simulink subsystem "Baseline"  (R2025b)
settings: Solver=VariableStepAuto  StartTime=0.0  StopTime=10.0  RelTol=1e-3
undefined symbols (not defined in the file): As_lat, As_lon, L1_LPF_bw, SimIn, SimPar, useL1
libraries: simulink_extras x23, ComponentsLib x11, matrix_library x2, AdaptiveLib x1, libAxisTransformations x1
settings Model: Creator=tbritton  LastModifiedBy=bullo
settings SolverCC: AlgebraicLoopSolver=TrustRegion
settings OptimizationCC: ReuseModelBlockBuffer=off
settings DebuggingCC: UnconnectedInputMsg=warning  UnconnectedOutputMsg=warning  UnconnectedLineMsg=warning
settings ModelReferenceCC: EnableRefExpFcnMdlSchedulingChecks=on
settings RTWCC: GPUComputeCapability=3.5  DLArmComputeVersion=19.05

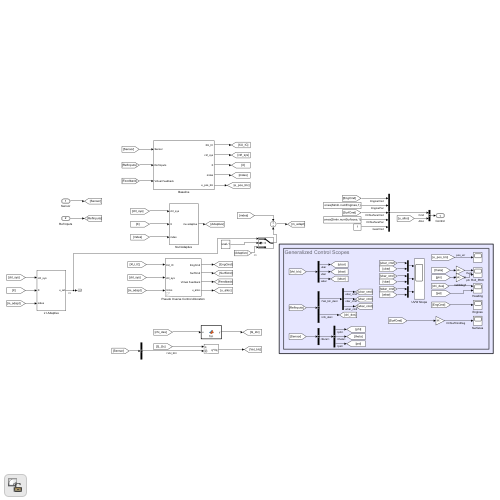
[thumbnail: Simulink's stored preview of the top-level diagram]
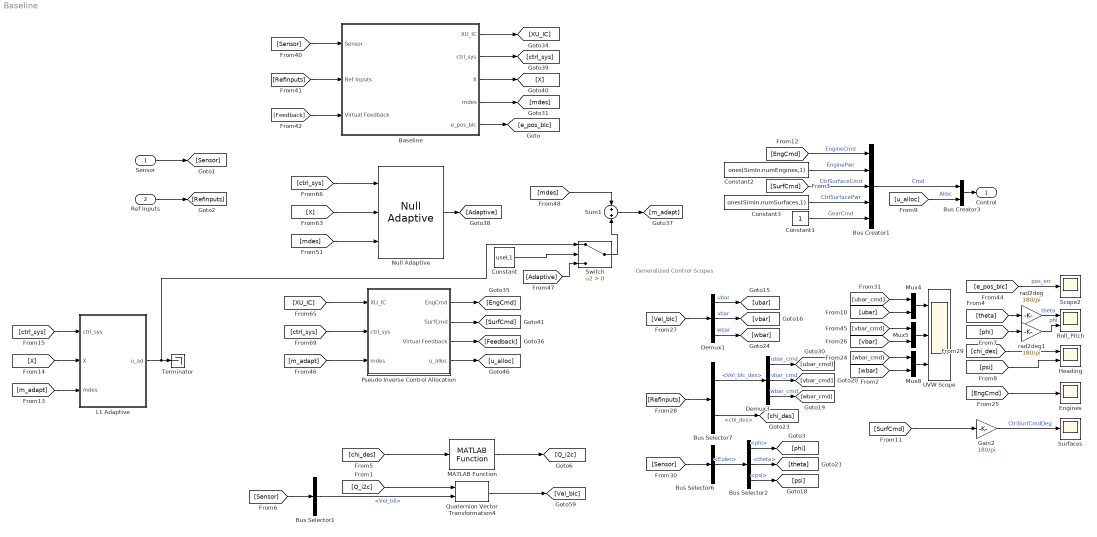
== system Baseline ==
  note: Generalized Control Scopes
  Sensor : Inport  OutDataTypeStr=Bus: SensorBus
  Ref Inputs : Inport  Port=2  OutDataTypeStr=Bus: BUS_REF_INPUT
  Baseline : Subsystem
      settings: LibrarySourceBlock=ControllersLib/Baseline
  Bus Creator1 : BusCreator  Inputs=5  OutDataTypeStr=Bus: BUS_CMD
  Bus Creator3 : BusCreator  Inputs=2
  Bus Selector1 : BusSelector  OutputSignals=Vel_bIi
  Bus Selector2 : BusSelector  OutputSignals=phi,theta,psi
  Bus Selector6 : BusSelector  OutputSignals=Euler
  Bus Selector7 : BusSelector  OutputSignals=Vel_bIc_des,chi_des
  Constant : Constant  Value=useL1
  Constant1 : Constant
  Constant2 : Constant  Value=ones(SimIn.numEngines,1)
  Constant3 : Constant  Value=ones(SimIn.numSurfaces,1)
  Demux1 : Demux  Outputs=3
  Demux3 : Demux  Outputs=3
  Engines : Scope
      settings: ActiveDisplayYMinimum=-12.285  ActiveDisplayYMaximum=110.56496
  Gain2 : Gain  Gain=180/pi
  Heading : Scope  NumInputPorts=2
      settings: ActiveDisplayYMinimum=-1.5E-19  ActiveDisplayYMaximum=1.3E-19  DataLoggingVariableName=ScopeData2
  L1 Adaptive : Subsystem
  MATLAB Function : ComponentsLib/ConvertToControlFrame/MATLAB Function  SystemSampleTime=-1  VariantActivationTime=update diagram  EmptyChoice=off  PassThrough=off  PassThroughVariantControl=(default)  EmptyChoiceVariantControl=(default)  AllowFlexibleInterface=on  Latency=0  AutoFrameSizeCalculation=off
      settings: SourceProductName=Components
  Mux4 : Mux  Inputs=2
  Mux5 : Mux  Inputs=2
  Mux8 : Mux  Inputs=2
  Null Adaptive : AdaptiveLib/Null Adaptive  SystemSampleTime=-1  VariantActivationTime=update diagram  EmptyChoice=off  PassThrough=off  PassThroughVariantControl=(default)  EmptyChoiceVariantControl=(default)  AllowFlexibleInterface=on  Latency=0  AutoFrameSizeCalculation=off
      settings: SourceProductName=Adaptive Augmentation
  Pseudo Inverse Control Allocation : Subsystem  AncestorBlock=AllocatorsLib/Pseudo Inverse Control Allocation
      settings: LibrarySourceBlock=AllocatorsLib/Pseudo Inverse Control Allocation
  Quaternion Vector Transformation4 : libAxisTransformations/Quaternion Vector Transformation  n=0
  Roll_Pitch : Scope  NumInputPorts=2
      settings: ActiveDisplayYMinimum=-0.0002  ActiveDisplayYMaximum=0.00013  DataLoggingVariableName=ScopeData3
  Scope2 : Scope
      settings: ActiveDisplayYMinimum=-0.07649  ActiveDisplayYMaximum=0.00878  DataLoggingVariableName=ScopeData4
  Sum1 : Sum
  Surfaces : Scope
      settings: ActiveDisplayYMinimum=-0.05034  ActiveDisplayYMaximum=0.00559  DataLoggingVariableName=ScopeData5
  Switch : Switch  Criteria=u2 > Threshold  SaturateOnIntegerOverflow=off  InputSameDT=off
  Terminator : Terminator
  UVW Scope : Scope  NumInputPorts=3
      settings: Title=UVW Commands vs Actual  ActiveDisplayYMinimum=-0.00149  ActiveDisplayYMaximum=0.01337  DataLoggingVariableName=ScopeData6
  rad2deg : Gain  Gain=180/pi
  rad2deg1 : Gain  Gain=180/pi
  Control : Outport  OutDataTypeStr=Bus: BUS_CONTROL  VectorParamsAs1DForOutWhenUnconnected=off
  wires:
  rad2deg1/1 -> Roll_Pitch/2  "phi"
  rad2deg/1 -> Roll_Pitch/1  "theta"
  Ref Inputs/1 -> [RefInputs]
  [u_alloc] -> Bus Creator3/2  "Alloc"
  Bus Creator3/1 -> Control/1
  Constant1/1 -> Bus Creator1/5  "GearCmd"
  [SurfCmd] -> Bus Creator1/3  "CtrlSurfaceCmd"
  Bus Creator1/1 -> Bus Creator3/1  "Cmd"
  Sensor/1 -> [Sensor]
  [EngCmd] -> Bus Creator1/1  "EngineCmd"
  Constant2/1 -> Bus Creator1/2  "EnginePwr"
  Constant3/1 -> Bus Creator1/4  "CtrlSurfacePwr"
  [Sensor] -> Baseline/1(Sensor)
  [RefInputs] -> Baseline/2(Ref Inputs)
  [Feedback] -> Baseline/3(Virtual Feedback)
  Baseline/4(mdes) -> [mdes]
  [m_adapt] -> Pseudo Inverse Control Allocation/3(mdes)
  Pseudo Inverse Control Allocation/3(Virtual Feedback) -> [Feedback]
  Baseline/1(XU_IC) -> [XU_IC]
  Pseudo Inverse Control Allocation/1(EngCmd) -> [EngCmd]
  [ctrl_sys] -> Null Adaptive/1
  [mdes] -> Null Adaptive/3
  [X] -> Null Adaptive/2
  Null Adaptive/1 -> [Adaptive]
  Baseline/2(ctrl_sys) -> [ctrl_sys]
  Baseline/3(X) -> [X]
  Sum1/1 -> [m_adapt]
  [mdes] -> Sum1/1
  Pseudo Inverse Control Allocation/2(SurfCmd) -> [SurfCmd]
  Pseudo Inverse Control Allocation/4(u_alloc) -> [u_alloc]
  [XU_IC] -> Pseudo Inverse Control Allocation/1(XU_IC)
  [ctrl_sys] -> Pseudo Inverse Control Allocation/2(ctrl_sys)
  Bus Selector1/1 -> Quaternion Vector Transformation4/2  "<Vel_bIi>"
  [Q_i2c] -> Quaternion Vector Transformation4/1
  [chi_des] -> MATLAB Function/1
  Quaternion Vector Transformation4/1 -> [Vel_bIc]
  MATLAB Function/1 -> [Q_i2c]
  [Sensor] -> Bus Selector1/1
  Demux1/3 -> [wbar]  "wbar"
  [wbar_cmd] -> Mux8/1
  Bus Selector7/2 -> [chi_des]  "<chi_des>"
  [Vel_bIc] -> Demux1/1
  Demux3/1 -> [ubar_cmd]  "ubar_cmd"
  Bus Selector7/1 -> Demux3/1  "<Vel_bIc_des>"
  [EngCmd] -> Engines/1
  Demux1/2 -> [vbar]  "vbar"
  [psi] -> Heading/2
  Bus Selector2/2 -> [theta]  "<theta>"
  [theta] -> rad2deg/1
  Gain2/1 -> Surfaces/1  "CtrlSurfCmdDeg"
  Bus Selector2/3 -> [psi]  "<psi>"
  Mux8/1 -> UVW Scope/3
  Bus Selector2/1 -> [phi]  "<phi>"
  Bus Selector6/1 -> Bus Selector2/1  "<Euler>"
  [e_pos_bIc] -> Scope2/1  "pos_err"
  Demux3/2 -> [vbar_cmd]  "vbar_cmd"
  [phi] -> rad2deg1/1
  [wbar] -> Mux8/2
  [RefInputs] -> Bus Selector7/1
  [Sensor] -> Bus Selector6/1
  [ubar] -> Mux4/2
  [chi_des] -> Heading/1
  [SurfCmd] -> Gain2/1
  [vbar] -> Mux5/2
  [ubar_cmd] -> Mux4/1
  [vbar_cmd] -> Mux5/1
  Mux5/1 -> UVW Scope/2
  Demux3/3 -> [wbar_cmd]  "wbar_cmd"
  Mux4/1 -> UVW Scope/1
  Demux1/1 -> [ubar]  "ubar"
  Baseline/5(e_pos_blc) -> [e_pos_bIc]
  [ctrl_sys] -> L1 Adaptive/1(ctrl_sys)
  [X] -> L1 Adaptive/2(X)
  [m_adapt] -> L1 Adaptive/3(mdes)
  Switch/1 -> Sum1/2
  L1 Adaptive/1(u_ad) -> Terminator/1, Switch/1
  [Adaptive] -> Switch/3
  Constant/1 -> Switch/2

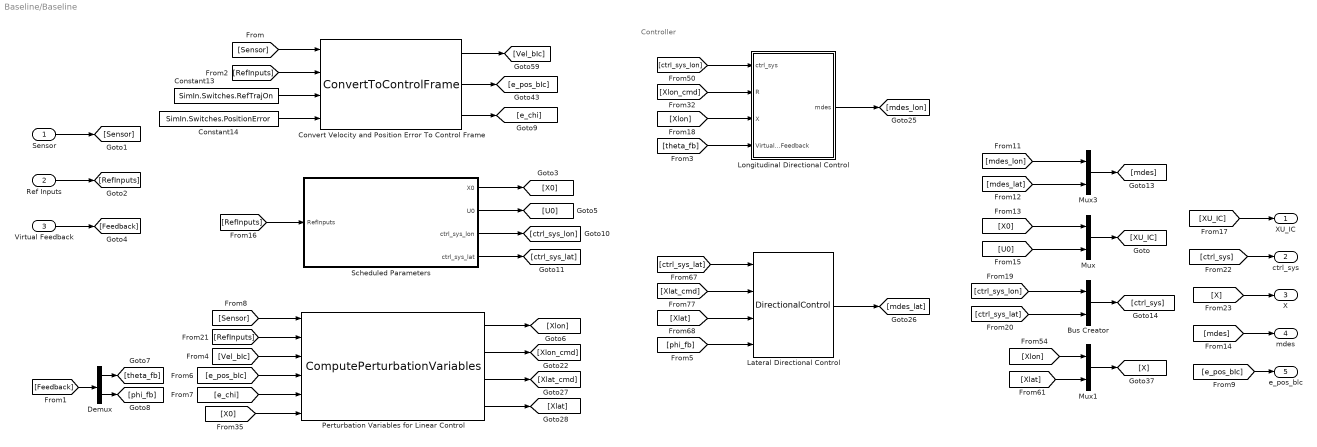
== system Baseline/Baseline ==
  note: Controller
  Sensor : Inport  OutDataTypeStr=Bus: SensorBus
  Ref Inputs : Inport  Port=2  OutDataTypeStr=Bus: BUS_REF_INPUT
  Virtual Feedback : Inport  Port=3
  Bus Creator : BusCreator  Inputs=2
  Constant13 : Constant  Value=SimIn.Switches.RefTrajOn
  Constant14 : Constant  Value=SimIn.Switches.PositionError
  Convert Velocity and Position Error To Control Frame : ComponentsLib/ConvertToControlFrame  SystemSampleTime=-1  VariantActivationTime=update diagram  EmptyChoice=off  PassThrough=off  PassThroughVariantControl=(default)  EmptyChoiceVariantControl=(default)  AllowFlexibleInterface=on  Latency=0  AutoFrameSizeCalculation=off
      link override delta_cos: Inputs=|++
      settings: SourceProductName=Components
  Demux : Demux  Outputs=2
  Lateral Directional Control : ComponentsLib/DirectionalControl  SystemSampleTime=-1  VariantActivationTime=update diagram  EmptyChoice=off  PassThrough=off  PassThroughVariantControl=(default)  EmptyChoiceVariantControl=(default)  AllowFlexibleInterface=on  Latency=0  AutoFrameSizeCalculation=off
      settings: SourceProductName=Components
  Longitudinal Directional Control : Subsystem  AncestorBlock=ComponentsLib/DirectionalControl
      settings: LibrarySourceBlock=ComponentsLib/DirectionalControl
  Mux : Mux  Inputs=2
  Mux1 : Mux  Inputs=2
  Mux3 : Mux  Inputs=2
  Perturbation Variables for Linear Control : ComponentsLib/ComputePerturbationVariables  SystemSampleTime=-1  VariantActivationTime=update diagram  EmptyChoice=off  PassThrough=off  PassThroughVariantControl=(default)  EmptyChoiceVariantControl=(default)  AllowFlexibleInterface=on  Latency=0  AutoFrameSizeCalculation=off
      settings: SourceProductName=Components
  Scheduled Parameters : Subsystem  AncestorBlock=ComponentsLib/FeedbackScheduling
      settings: LibrarySourceBlock=ComponentsLib/FeedbackScheduling
  XU_IC : Outport
  ctrl_sys : Outport  Port=2
  X : Outport  Port=3
  mdes : Outport  Port=4
  e_pos_blc : Outport  Port=5
  wires:
  [mdes_lat] -> Mux3/2
  [e_pos_bIc] -> e_pos_blc/1
  [X0] -> Perturbation Variables for Linear Control/6
  Perturbation Variables for Linear Control/1 -> [Xlon]
  [Sensor] -> Perturbation Variables for Linear Control/1
  Perturbation Variables for Linear Control/3 -> [Xlat_cmd]
  Sensor/1 -> [Sensor]
  Scheduled Parameters/1(X0) -> [X0]
  Ref Inputs/1 -> [RefInputs]
  [RefInputs] -> Convert Velocity and Position Error To Control Frame/2
  Convert Velocity and Position Error To Control Frame/1 -> [Vel_bIc]
  Convert Velocity and Position Error To Control Frame/2 -> [e_pos_bIc]
  Scheduled Parameters/3(ctrl_sys_lon) -> [ctrl_sys_lon]
  [e_pos_bIc] -> Perturbation Variables for Linear Control/4
  Perturbation Variables for Linear Control/4 -> [Xlat]
  [RefInputs] -> Scheduled Parameters/1(RefInputs)
  Perturbation Variables for Linear Control/2 -> [Xlon_cmd]
  Convert Velocity and Position Error To Control Frame/3 -> [e_chi]
  [Sensor] -> Convert Velocity and Position Error To Control Frame/1
  [Vel_bIc] -> Perturbation Variables for Linear Control/3
  Constant13/1 -> Convert Velocity and Position Error To Control Frame/3
  [RefInputs] -> Perturbation Variables for Linear Control/2
  Constant14/1 -> Convert Velocity and Position Error To Control Frame/4
  [e_chi] -> Perturbation Variables for Linear Control/5
  Scheduled Parameters/2(U0) -> [U0]
  Scheduled Parameters/4(ctrl_sys_lat) -> [ctrl_sys_lat]
  [Xlon_cmd] -> Longitudinal Directional Control/2(R)
  Lateral Directional Control/1 -> [mdes_lat]
  [ctrl_sys_lat] -> Lateral Directional Control/1
  [ctrl_sys_lon] -> Longitudinal Directional Control/1(ctrl_sys)
  Longitudinal Directional Control/1(mdes) -> [mdes_lon]
  [Xlat] -> Lateral Directional Control/3
  [Xlon] -> Longitudinal Directional Control/3(X)
  [Xlat_cmd] -> Lateral Directional Control/2
  Virtual Feedback/1 -> [Feedback]
  [Feedback] -> Demux/1
  Demux/2 -> [phi_fb]
  Demux/1 -> [theta_fb]
  [theta_fb] -> Longitudinal Directional Control/4(Virtual Feedback)
  [phi_fb] -> Lateral Directional Control/4
  [mdes_lon] -> Mux3/1
  Mux3/1 -> [mdes]
  [mdes] -> mdes/1
  [X0] -> Mux/1
  [U0] -> Mux/2
  Mux/1 -> [XU_IC]
  [XU_IC] -> XU_IC/1
  [ctrl_sys_lon] -> Bus Creator/1
  [ctrl_sys_lat] -> Bus Creator/2
  Bus Creator/1 -> [ctrl_sys]
  [ctrl_sys] -> ctrl_sys/1
  Mux1/1 -> [X]
  [Xlon] -> Mux1/1
  [Xlat] -> Mux1/2
  [X] -> X/1

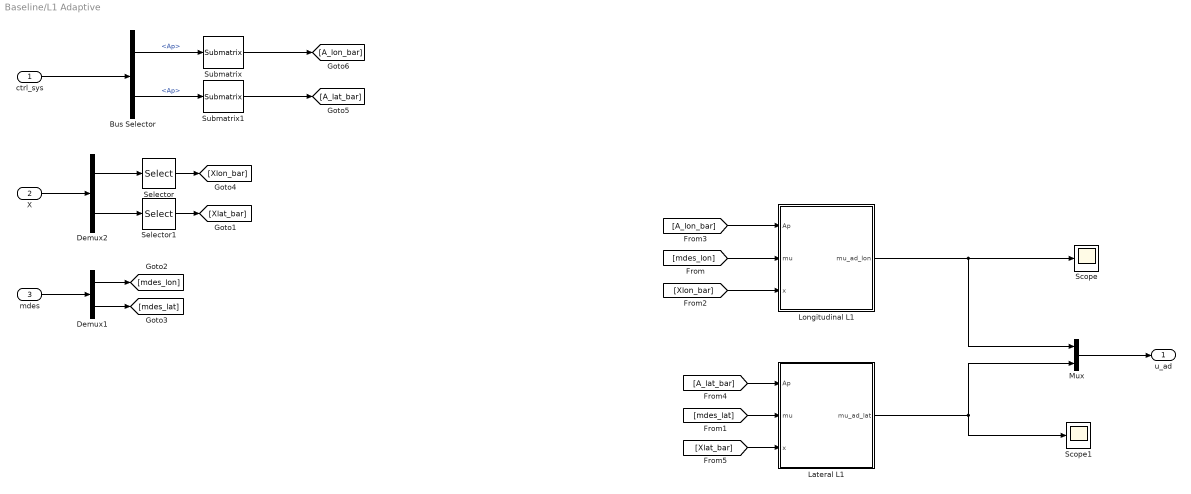
== system Baseline/L1 Adaptive ==
  ctrl_sys : Inport
  X : Inport  Port=2
  mdes : Inport  Port=3
  Bus Selector : BusSelector  OutputSignals=ctrl_sys_lon.Ap,ctrl_sys_lat.Ap
  Demux1 : Demux  Outputs=2
  Demux2 : Demux  Outputs=2
  Lateral L1 : Subsystem
  Longitudinal L1 : Subsystem
  Mux : Mux  Inputs=2
  Scope : Scope
      settings: ActiveDisplayYMinimum=-28.653376780680318  ActiveDisplayYMaximum=12.641940394712167  DataLoggingVariableName=ScopeData11
  Scope1 : Scope
      settings: ActiveDisplayYMinimum=-8.3781527224197525  ActiveDisplayYMaximum=15.883080645115539  DataLoggingVariableName=ScopeData12
  Selector : Selector  InputPortWidth=4  IndexOptions=Index vector (dialog)  Indices=[1:3]  OutputSizes=1
  Selector1 : Selector  InputPortWidth=4  IndexOptions=Index vector (dialog)  Indices=[1:3]  OutputSizes=1
  Submatrix : matrix_library/Submatrix  RowSpan=Range of rows  RowStartMode=First  RowStartIndex=1  RowEndMode=Index  RowEndIndex=3  ColSpan=Range of columns  ColStartMode=First  ColStartIndex=1  ColEndMode=Index  ColEndIndex=3
  Submatrix1 : matrix_library/Submatrix  RowSpan=Range of rows  RowStartMode=First  RowStartIndex=1  RowEndMode=Index  RowEndIndex=3  ColSpan=Range of columns  ColStartMode=First  ColStartIndex=1  ColEndMode=Index  ColEndIndex=3
  u_ad : Outport
  wires:
  [A_lat_bar] -> Lateral L1/1(Ap)
  [mdes_lat] -> Lateral L1/2(mu)
  Lateral L1/1(mu_ad_lat) -> Mux/2, Scope1/1
  [Xlat_bar] -> Lateral L1/3(x)
  [A_lon_bar] -> Longitudinal L1/1(Ap)
  Submatrix/1 -> [A_lon_bar]
  Submatrix1/1 -> [A_lat_bar]
  Bus Selector/2 -> Submatrix1/1  "<Ap>"
  Selector1/1 -> [Xlat_bar]
  [Xlon_bar] -> Longitudinal L1/3(x)
  Selector/1 -> [Xlon_bar]
  Mux/1 -> u_ad/1
  [mdes_lon] -> Longitudinal L1/2(mu)
  Longitudinal L1/1(mu_ad_lon) -> Scope/1, Mux/1
  Demux2/2 -> Selector1/1
  Demux2/1 -> Selector/1
  Bus Selector/1 -> Submatrix/1  "<Ap>"
  Demux1/1 -> [mdes_lon]
  Demux1/2 -> [mdes_lat]
  mdes/1 -> Demux1/1
  X/1 -> Demux2/1
  ctrl_sys/1 -> Bus Selector/1

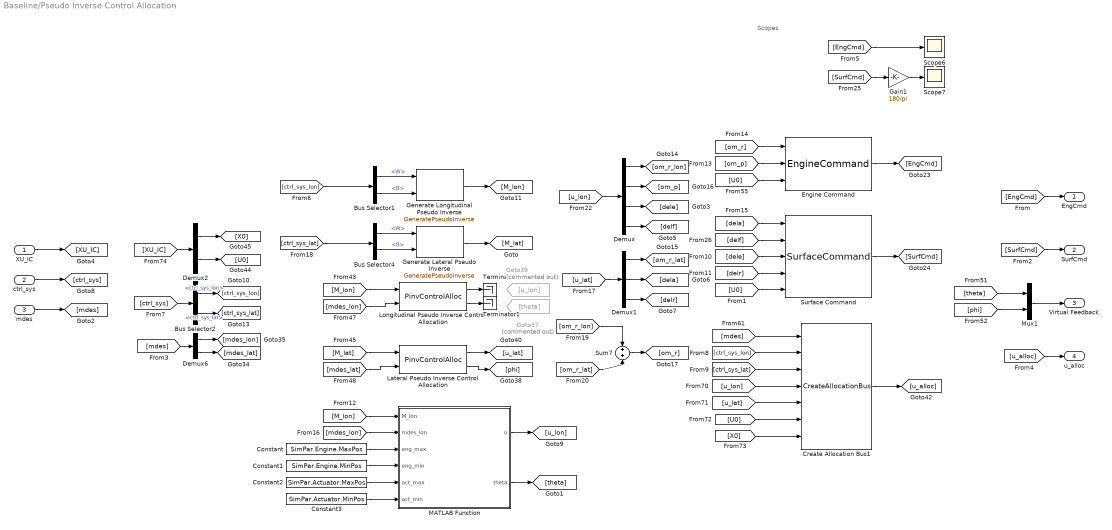
== system Baseline/Pseudo Inverse Control Allocation ==
  note: Scopes
  XU_IC : Inport
  ctrl_sys : Inport  Port=2
  mdes : Inport  Port=3
  Bus Selector1 : BusSelector  OutputSignals=W,B
  Bus Selector2 : BusSelector  OutputSignals=ctrl_sys_lon,ctrl_sys_lat
  Bus Selector4 : BusSelector  OutputSignals=W,B
  Constant : Constant  Value=SimPar.Engine.MaxPos
  Constant1 : Constant  Value=SimPar.Engine.MinPos
  Constant2 : Constant  Value=SimPar.Actuator.MaxPos
  Constant3 : Constant  Value=SimPar.Actuator.MinPos
  Create Allocation Bus1 : ComponentsLib/CreateAllocationBus  SystemSampleTime=-1  VariantActivationTime=update diagram  EmptyChoice=off  PassThrough=off  PassThroughVariantControl=(default)  EmptyChoiceVariantControl=(default)  AllowFlexibleInterface=on  Latency=0  AutoFrameSizeCalculation=off
      settings: SourceProductName=Components
  Demux : Demux  Outputs=[8 1 1 1]
  Demux1 : Demux  Outputs=[8 1 1]
  Demux2 : Demux  Outputs=[12 13]
  Demux6 : Demux  Outputs=[3 3]
  Engine Command : ComponentsLib/EngineCommand  SystemSampleTime=-1  VariantActivationTime=update diagram  EmptyChoice=off  PassThrough=off  PassThroughVariantControl=(default)  EmptyChoiceVariantControl=(default)  AllowFlexibleInterface=on  Latency=0  AutoFrameSizeCalculation=off
      settings: SourceProductName=Components
  Gain1 : Gain  Gain=180/pi
  Generate Lateral Pseudo Inverse : ComponentsLib/GeneratePseudoInverse  SystemSampleTime=-1  VariantActivationTime=update diagram  EmptyChoice=off  PassThrough=off  PassThroughVariantControl=(default)  EmptyChoiceVariantControl=(default)  AllowFlexibleInterface=on  Latency=0  AutoFrameSizeCalculation=off
      settings: SourceProductName=Components
  Generate Longitudinal Pseudo Inverse : ComponentsLib/GeneratePseudoInverse  SystemSampleTime=-1  VariantActivationTime=update diagram  EmptyChoice=off  PassThrough=off  PassThroughVariantControl=(default)  EmptyChoiceVariantControl=(default)  AllowFlexibleInterface=on  Latency=0  AutoFrameSizeCalculation=off
      settings: SourceProductName=Components
  Goto37 : Goto  Commented=on  GotoTag=theta
  Goto39 : Goto  Commented=on  GotoTag=u_lon
  Lateral Pseudo Inverse Control Allocation : ComponentsLib/PinvControlAlloc  SystemSampleTime=-1  VariantActivationTime=update diagram  EmptyChoice=off  PassThrough=off  PassThroughVariantControl=(default)  EmptyChoiceVariantControl=(default)  AllowFlexibleInterface=on  Latency=0  AutoFrameSizeCalculation=off
      settings: SourceProductName=Components
  Longitudinal Pseudo Inverse Control Allocation : ComponentsLib/PinvControlAlloc  SystemSampleTime=-1  VariantActivationTime=update diagram  EmptyChoice=off  PassThrough=off  PassThroughVariantControl=(default)  EmptyChoiceVariantControl=(default)  AllowFlexibleInterface=on  Latency=0  AutoFrameSizeCalculation=off
      settings: SourceProductName=Components
  MATLAB Function : MATLAB Function  TreatAsAtomicUnit=on
  Mux1 : Mux  Inputs=2
  Scope6 : Scope
      settings: ActiveDisplayYMinimum=-43.75112  ActiveDisplayYMaximum=393.75013  DataLoggingVariableName=ScopeData11
  Scope7 : Scope
      settings: ActiveDisplayYMinimum=-36.29377  ActiveDisplayYMaximum=26.64394  DataLoggingVariableName=ScopeData12
  Sum7 : Sum
  Surface Command : ComponentsLib/SurfaceCommand  SystemSampleTime=-1  VariantActivationTime=update diagram  EmptyChoice=off  PassThrough=off  PassThroughVariantControl=(default)  EmptyChoiceVariantControl=(default)  AllowFlexibleInterface=on  Latency=0  AutoFrameSizeCalculation=off
      settings: SourceProductName=Components
  Terminator : Terminator
  Terminator1 : Terminator
  EngCmd : Outport
  SurfCmd : Outport  Port=2
  Virtual Feedback : Outport  Port=3
  u_alloc : Outport  Port=4
  wires:
  Lateral Pseudo Inverse Control Allocation/2 -> [phi]
  Longitudinal Pseudo Inverse Control Allocation/1 -> Terminator/1
  [theta] -> Mux1/1
  [mdes_lat] -> Lateral Pseudo Inverse Control Allocation/2
  [phi] -> Mux1/2
  [mdes_lon] -> Longitudinal Pseudo Inverse Control Allocation/2
  Lateral Pseudo Inverse Control Allocation/1 -> [u_lat]
  Longitudinal Pseudo Inverse Control Allocation/2 -> Terminator1/1
  Mux1/1 -> Virtual Feedback/1
  [M_lon] -> Longitudinal Pseudo Inverse Control Allocation/1
  [M_lat] -> Lateral Pseudo Inverse Control Allocation/1
  Demux/3 -> [dele]
  Demux/2 -> [om_p]
  [u_lat] -> Demux1/1
  [om_r_lat] -> Sum7/2
  [om_r_lon] -> Sum7/1
  Sum7/1 -> [om_r]
  [u_lon] -> Demux/1
  Demux1/2 -> [dela]
  Demux1/1 -> [om_r_lat]
  Demux/1 -> [om_r_lon]
  Demux/4 -> [delf]
  Demux1/3 -> [delr]
  Engine Command/1 -> [EngCmd]
  Surface Command/1 -> [SurfCmd]
  [U0] -> Engine Command/3
  [dele] -> Surface Command/3
  [delf] -> Surface Command/2
  [delr] -> Surface Command/4
  [om_p] -> Engine Command/2
  [om_r] -> Engine Command/1
  [U0] -> Surface Command/5
  [dela] -> Surface Command/1
  [EngCmd] -> EngCmd/1
  [SurfCmd] -> SurfCmd/1
  Demux2/2 -> [U0]
  [U0] -> Create Allocation Bus1/6
  [u_lon] -> Create Allocation Bus1/4
  Create Allocation Bus1/1 -> [u_alloc]
  [u_lat] -> Create Allocation Bus1/5
  [XU_IC] -> Demux2/1
  [X0] -> Create Allocation Bus1/7
  Demux2/1 -> [X0]
  [mdes] -> Create Allocation Bus1/1
  Demux6/2 -> [mdes_lat]
  Demux6/1 -> [mdes_lon]
  [mdes] -> Demux6/1
  mdes/1 -> [mdes]
  XU_IC/1 -> [XU_IC]
  ctrl_sys/1 -> [ctrl_sys]
  [u_alloc] -> u_alloc/1
  Gain1/1 -> Scope7/1
  [SurfCmd] -> Gain1/1
  [EngCmd] -> Scope6/1
  [ctrl_sys_lat] -> Bus Selector4/1
  Bus Selector1/1 -> Generate Longitudinal Pseudo Inverse/1  "<W>"
  [ctrl_sys_lon] -> Bus Selector1/1
  Generate Longitudinal Pseudo Inverse/1 -> [M_lon]
  Bus Selector4/1 -> Generate Lateral Pseudo Inverse/1  "<W>"
  Generate Lateral Pseudo Inverse/1 -> [M_lat]
  Bus Selector4/2 -> Generate Lateral Pseudo Inverse/2  "<B>"
  Bus Selector1/2 -> Generate Longitudinal Pseudo Inverse/2  "<B>"
  [ctrl_sys] -> Bus Selector2/1
  Bus Selector2/1 -> [ctrl_sys_lon]  "<ctrl_sys_lon>"
  Bus Selector2/2 -> [ctrl_sys_lat]  "<ctrl_sys_lat>"
  [ctrl_sys_lon] -> Create Allocation Bus1/2
  [ctrl_sys_lat] -> Create Allocation Bus1/3
  [M_lon] -> MATLAB Function/1(M_lon)
  [mdes_lon] -> MATLAB Function/2(mdes_lon)
  MATLAB Function/1(u) -> [u_lon]
  MATLAB Function/2(theta) -> [theta]
  Constant3/1 -> MATLAB Function/6(act_min)
  Constant2/1 -> MATLAB Function/5(act_max)
  Constant1/1 -> MATLAB Function/4(eng_min)
  Constant/1 -> MATLAB Function/3(eng_max)

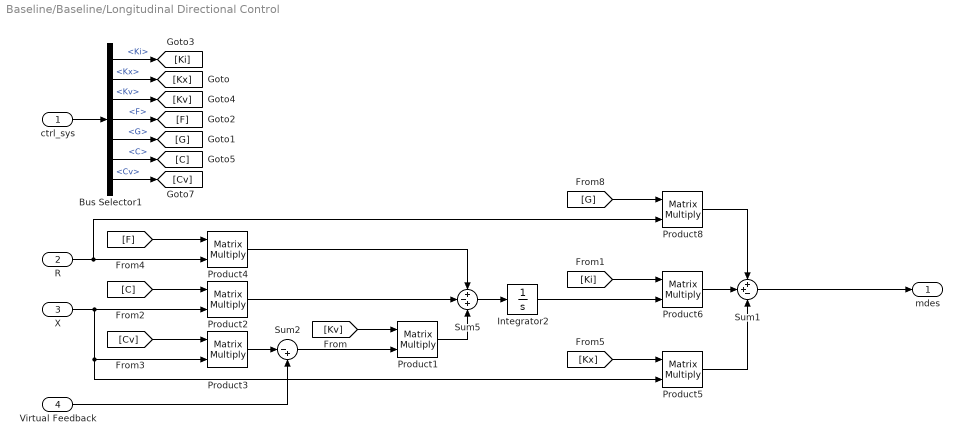
== system Baseline/Baseline/Longitudinal Directional Control ==
  ctrl_sys : Inport
  R : Inport  Port=2
  X : Inport  Port=3
  Virtual Feedback : Inport  Port=4
  Bus Selector1 : BusSelector  OutputSignals=Ki,Kx,Kv,F,G,C,Cv
  Integrator2 : Integrator  UpperSaturationLimit=[10 10 1]  LowerSaturationLimit=[-10 -10 -1]
  Product{1..6,8} (7 alike) : Product  Multiplication=Matrix(*)
  Sum1 : Sum  Inputs=++-
  Sum2 : Sum  Inputs=|-+
  Sum5 : Sum  Inputs=+-+
  mdes : Outport
  wires:
  Sum1/1 -> mdes/1
  X/1 -> Product2/2, Product3/2, Product5/2
  [C] -> Product2/1
  Product2/1 -> Sum5/2
  R/1 -> Product8/2, Product4/2
  Sum5/1 -> Integrator2/1
  ctrl_sys/1 -> Bus Selector1/1
  [Cv] -> Product3/1
  Product3/1 -> Sum2/1
  Integrator2/1 -> Product6/2
  Sum2/1 -> Product1/2
  [Kv] -> Product1/1
  Product1/1 -> Sum5/3
  [Ki] -> Product6/1
  Product6/1 -> Sum1/2
  [Kx] -> Product5/1
  Product5/1 -> Sum1/3
  [F] -> Product4/1
  Product4/1 -> Sum5/1
  Product8/1 -> Sum1/1
  [G] -> Product8/1
  Virtual Feedback/1 -> Sum2/2
  Bus Selector1/7 -> [Cv]  "<Cv>"
  Bus Selector1/6 -> [C]  "<C>"
  Bus Selector1/5 -> [G]  "<G>"
  Bus Selector1/4 -> [F]  "<F>"
  Bus Selector1/3 -> [Kv]  "<Kv>"
  Bus Selector1/2 -> [Kx]  "<Kx>"
  Bus Selector1/1 -> [Ki]  "<Ki>"

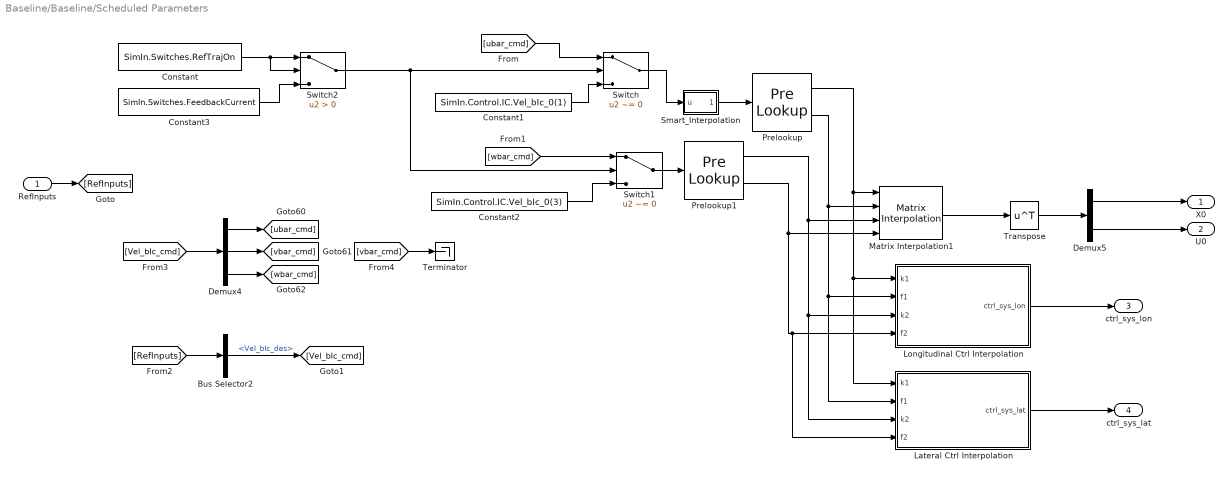
== system Baseline/Baseline/Scheduled Parameters ==
  RefInputs : Inport  OutDataTypeStr=Bus: BUS_REF_INPUT
  Bus Selector2 : BusSelector  OutputSignals=Vel_bIc_des
  Constant : Constant  Value=SimIn.Switches.RefTrajOn
  Constant1 : Constant  Value=SimIn.Control.IC.Vel_bIc_0(1)
  Constant2 : Constant  Value=SimIn.Control.IC.Vel_bIc_0(3)
  Constant3 : Constant  Value=SimIn.Switches.FeedbackCurrent
  Demux4 : Demux  Outputs=3
  Demux5 : Demux  Outputs=[12 13]
  Lateral Ctrl Interpolation : Subsystem
  Longitudinal Ctrl Interpolation : Subsystem
  Matrix Interpolation1 : simulink_extras/Additional Lookup Tables/Matrix Interpolation  InterpMethod=Linear  ExtrapMethod=Clip  InterpolateDimension=2  TableData=SimIn.Control.trim.XU0_interp  SimulateUsing=Code generation
  Prelookup : PreLookup  BreakpointsData=SimIn.Control.trim.UH
  Prelookup1 : PreLookup  BreakpointsData=SimIn.Control.trim.WH
  Smart_Interpolation : MATLAB Function  TreatAsAtomicUnit=on
  Switch : Switch  Criteria=u2 ~= 0  SaturateOnIntegerOverflow=off  InputSameDT=off
  Switch1 : Switch  Criteria=u2 ~= 0  SaturateOnIntegerOverflow=off  InputSameDT=off
  Switch2 : Switch  Criteria=u2 > Threshold  SaturateOnIntegerOverflow=off  InputSameDT=off
  Terminator : Terminator
  Transpose : Math  Operator=transpose
  X0 : Outport
  U0 : Outport  Port=2
  ctrl_sys_lon : Outport  Port=3
  ctrl_sys_lat : Outport  Port=4
  wires:
  Prelookup/1 -> Lateral Ctrl Interpolation/1(k1), Longitudinal Ctrl Interpolation/1(k1), Matrix Interpolation1/1
  Prelookup/2 -> Matrix Interpolation1/2, Lateral Ctrl Interpolation/2(f1), Longitudinal Ctrl Interpolation/2(f1)
  Smart_Interpolation/1(u_out) -> Prelookup/1
  Switch/1 -> Smart_Interpolation/1(u)
  Constant3/1 -> Switch2/3
  Constant/1 -> Switch2/2, Switch2/1
  Switch2/1 -> Switch/2, Switch1/2
  Constant2/1 -> Switch1/3
  Switch1/1 -> Prelookup1/1
  Constant1/1 -> Switch/3
  Longitudinal Ctrl Interpolation/1(ctrl_sys_lon) -> ctrl_sys_lon/1
  Lateral Ctrl Interpolation/1(ctrl_sys_lat) -> ctrl_sys_lat/1
  Prelookup1/2 -> Matrix Interpolation1/4, Lateral Ctrl Interpolation/4(f2), Longitudinal Ctrl Interpolation/4(f2)
  Prelookup1/1 -> Matrix Interpolation1/3, Lateral Ctrl Interpolation/3(k2), Longitudinal Ctrl Interpolation/3(k2)
  Demux5/2 -> U0/1
  Demux5/1 -> X0/1
  Transpose/1 -> Demux5/1
  Matrix Interpolation1/1 -> Transpose/1
  Demux4/1 -> [ubar_cmd]
  Demux4/3 -> [wbar_cmd]
  Demux4/2 -> [vbar_cmd]
  [Vel_bIc_cmd] -> Demux4/1
  RefInputs/1 -> [RefInputs]
  [ubar_cmd] -> Switch/1
  [RefInputs] -> Bus Selector2/1
  Bus Selector2/1 -> [Vel_bIc_cmd]  "<Vel_bIc_des>"
  [vbar_cmd] -> Terminator/1
  [wbar_cmd] -> Switch1/1

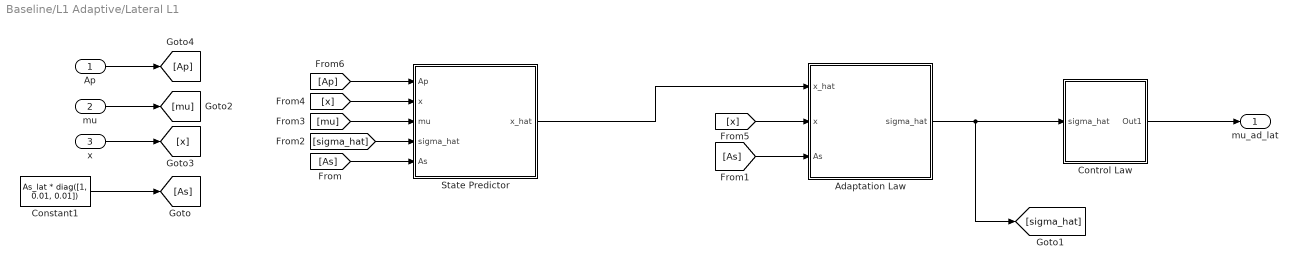
== system Baseline/L1 Adaptive/Lateral L1 ==
  Ap : Inport
  mu : Inport  Port=2
  x : Inport  Port=3
  Adaptation Law : Subsystem
  Constant1 : Constant  Value=As_lat * diag([1, 0.01, 0.01])
  Control Law : Subsystem
  State Predictor : Subsystem
  mu_ad_lat : Outport
  wires:
  Ap/1 -> [Ap]
  State Predictor/1(x_hat) -> Adaptation Law/1(x_hat)
  Control Law/1(Out1) -> mu_ad_lat/1
  x/1 -> [x]
  Adaptation Law/1(sigma_hat) -> [sigma_hat], Control Law/1(sigma_hat)
  Constant1/1 -> [As]
  [As] -> State Predictor/5(As)
  [As] -> Adaptation Law/3(As)
  [sigma_hat] -> State Predictor/4(sigma_hat)
  mu/1 -> [mu]
  [mu] -> State Predictor/3(mu)
  [x] -> State Predictor/2(x)
  [x] -> Adaptation Law/2(x)
  [Ap] -> State Predictor/1(Ap)

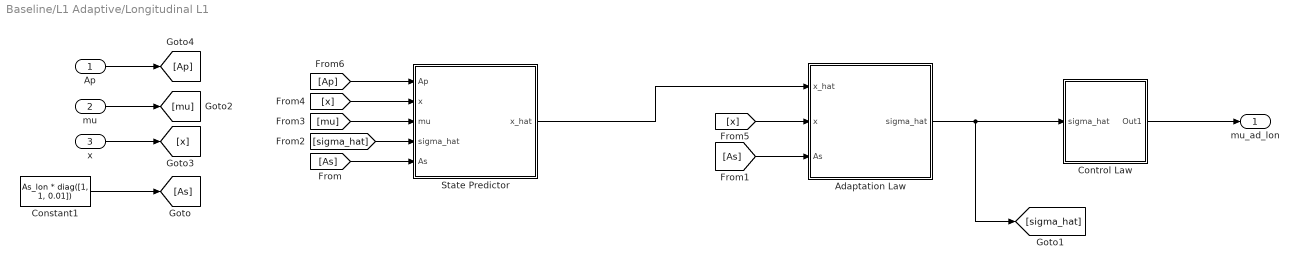
== system Baseline/L1 Adaptive/Longitudinal L1 ==
  Ap : Inport
  mu : Inport  Port=2
  x : Inport  Port=3
  Adaptation Law : Subsystem
  Constant1 : Constant  Value=As_lon * diag([1, 1, 0.01])
  Control Law : Subsystem
  State Predictor : Subsystem
  mu_ad_lon : Outport
  wires:
  x/1 -> [x]
  Ap/1 -> [Ap]
  mu/1 -> [mu]
  Constant1/1 -> [As]
  [Ap] -> State Predictor/1(Ap)
  [x] -> Adaptation Law/2(x)
  [x] -> State Predictor/2(x)
  [mu] -> State Predictor/3(mu)
  [As] -> State Predictor/5(As)
  [sigma_hat] -> State Predictor/4(sigma_hat)
  Adaptation Law/1(sigma_hat) -> [sigma_hat], Control Law/1(sigma_hat)
  [As] -> Adaptation Law/3(As)
  State Predictor/1(x_hat) -> Adaptation Law/1(x_hat)
  Control Law/1(Out1) -> mu_ad_lon/1

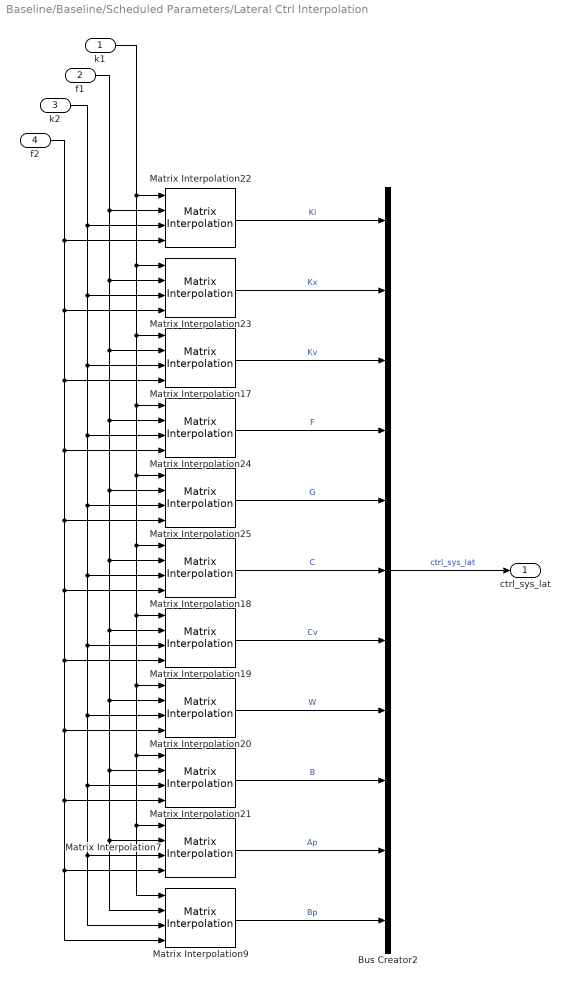
== system Baseline/Baseline/Scheduled Parameters/Lateral Ctrl Interpolation ==
  k1 : Inport
  f1 : Inport  Port=2
  k2 : Inport  Port=3
  f2 : Inport  Port=4
  Bus Creator2 : BusCreator  Inputs=11
  Matrix Interpolation17 : simulink_extras/Additional Lookup Tables/Matrix Interpolation  InterpMethod=Linear  ExtrapMethod=Clip  InterpolateDimension=2  TableData=SimIn.Control.trim.Kv_lat_interp  SimulateUsing=Code generation
  Matrix Interpolation18 : simulink_extras/Additional Lookup Tables/Matrix Interpolation  InterpMethod=Linear  ExtrapMethod=Clip  InterpolateDimension=2  TableData=SimIn.Control.trim.C_lat_interp  SimulateUsing=Code generation
  Matrix Interpolation19 : simulink_extras/Additional Lookup Tables/Matrix Interpolation  InterpMethod=Linear  ExtrapMethod=Clip  InterpolateDimension=2  TableData=SimIn.Control.trim.Cv_lat_interp  SimulateUsing=Code generation
  Matrix Interpolation20 : simulink_extras/Additional Lookup Tables/Matrix Interpolation  InterpMethod=Linear  ExtrapMethod=Clip  InterpolateDimension=2  TableData=SimIn.Control.trim.W_lat_interp  SimulateUsing=Code generation
  Matrix Interpolation21 : simulink_extras/Additional Lookup Tables/Matrix Interpolation  InterpMethod=Linear  ExtrapMethod=Clip  InterpolateDimension=2  TableData=SimIn.Control.trim.B_lat_interp  SimulateUsing=Code generation
  Matrix Interpolation22 : simulink_extras/Additional Lookup Tables/Matrix Interpolation  InterpMethod=Linear  ExtrapMethod=Clip  InterpolateDimension=2  TableData=SimIn.Control.trim.Ki_lat_interp  SimulateUsing=Code generation
  Matrix Interpolation23 : simulink_extras/Additional Lookup Tables/Matrix Interpolation  InterpMethod=Linear  ExtrapMethod=Clip  InterpolateDimension=2  TableData=SimIn.Control.trim.Kx_lat_interp  SimulateUsing=Code generation
  Matrix Interpolation24 : simulink_extras/Additional Lookup Tables/Matrix Interpolation  InterpMethod=Linear  ExtrapMethod=Clip  InterpolateDimension=2  TableData=SimIn.Control.trim.F_lat_interp  SimulateUsing=Code generation
  Matrix Interpolation25 : simulink_extras/Additional Lookup Tables/Matrix Interpolation  InterpMethod=Linear  ExtrapMethod=Clip  InterpolateDimension=2  TableData=SimIn.Control.trim.G_lat_interp  SimulateUsing=Code generation
  Matrix Interpolation7 : simulink_extras/Additional Lookup Tables/Matrix Interpolation  InterpMethod=Linear  ExtrapMethod=Clip  InterpolateDimension=2  TableData=SimIn.Control.trim.Ap_lat_interp  SimulateUsing=Code generation
  Matrix Interpolation9 : simulink_extras/Additional Lookup Tables/Matrix Interpolation  InterpMethod=Linear  ExtrapMethod=Clip  InterpolateDimension=2  TableData=SimIn.Control.trim.Bp_lat_interp  SimulateUsing=Code generation
  ctrl_sys_lat : Outport
  wires:
  Bus Creator2/1 -> ctrl_sys_lat/1  "ctrl_sys_lat"
  Matrix Interpolation7/1 -> Bus Creator2/10  "Ap"
  Matrix Interpolation21/1 -> Bus Creator2/9  "B"
  Matrix Interpolation24/1 -> Bus Creator2/4  "F"
  Matrix Interpolation25/1 -> Bus Creator2/5  "G"
  Matrix Interpolation9/1 -> Bus Creator2/11  "Bp"
  Matrix Interpolation23/1 -> Bus Creator2/2  "Kx"
  Matrix Interpolation19/1 -> Bus Creator2/7  "Cv"
  Matrix Interpolation18/1 -> Bus Creator2/6  "C"
  Matrix Interpolation17/1 -> Bus Creator2/3  "Kv"
  Matrix Interpolation22/1 -> Bus Creator2/1  "Ki"
  f1/1 -> Matrix Interpolation9/2, Matrix Interpolation7/2, Matrix Interpolation21/2, Matrix Interpolation20/2, Matrix Interpolation19/2, Matrix Interpolation18/2, Matrix Interpolation25/2, Matrix Interpolation24/2, Matrix Interpolation17/2, Matrix Interpolation23/2, Matrix Interpolation22/2
  f2/1 -> Matrix Interpolation9/4, Matrix Interpolation7/4, Matrix Interpolation21/4, Matrix Interpolation20/4, Matrix Interpolation19/4, Matrix Interpolation18/4, Matrix Interpolation25/4, Matrix Interpolation24/4, Matrix Interpolation17/4, Matrix Interpolation23/4, Matrix Interpolation22/4
  Matrix Interpolation20/1 -> Bus Creator2/8  "W"
  k2/1 -> Matrix Interpolation9/3, Matrix Interpolation7/3, Matrix Interpolation21/3, Matrix Interpolation20/3, Matrix Interpolation19/3, Matrix Interpolation18/3, Matrix Interpolation25/3, Matrix Interpolation24/3, Matrix Interpolation17/3, Matrix Interpolation23/3, Matrix Interpolation22/3
  k1/1 -> Matrix Interpolation24/1, Matrix Interpolation20/1, Matrix Interpolation7/1, Matrix Interpolation9/1, Matrix Interpolation21/1, Matrix Interpolation19/1, Matrix Interpolation18/1, Matrix Interpolation25/1, Matrix Interpolation17/1, Matrix Interpolation23/1, Matrix Interpolation22/1

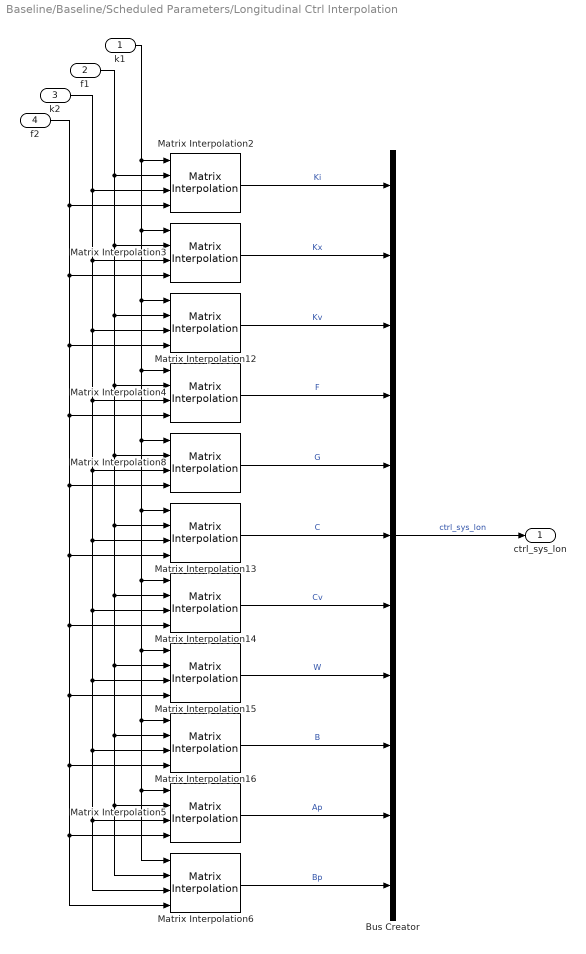
== system Baseline/Baseline/Scheduled Parameters/Longitudinal Ctrl Interpolation ==
  k1 : Inport
  f1 : Inport  Port=2
  k2 : Inport  Port=3
  f2 : Inport  Port=4
  Bus Creator : BusCreator  Inputs=11
  Matrix Interpolation12 : simulink_extras/Additional Lookup Tables/Matrix Interpolation  InterpMethod=Linear  ExtrapMethod=Clip  InterpolateDimension=2  TableData=SimIn.Control.trim.Kv_lon_interp  SimulateUsing=Code generation
  Matrix Interpolation13 : simulink_extras/Additional Lookup Tables/Matrix Interpolation  InterpMethod=Linear  ExtrapMethod=Clip  InterpolateDimension=2  TableData=SimIn.Control.trim.C_lon_interp  SimulateUsing=Code generation
  Matrix Interpolation14 : simulink_extras/Additional Lookup Tables/Matrix Interpolation  InterpMethod=Linear  ExtrapMethod=Clip  InterpolateDimension=2  TableData=SimIn.Control.trim.Cv_lon_interp  SimulateUsing=Code generation
  Matrix Interpolation15 : simulink_extras/Additional Lookup Tables/Matrix Interpolation  InterpMethod=Linear  ExtrapMethod=Clip  InterpolateDimension=2  TableData=SimIn.Control.trim.W_lon_interp  SimulateUsing=Code generation
  Matrix Interpolation16 : simulink_extras/Additional Lookup Tables/Matrix Interpolation  InterpMethod=Linear  ExtrapMethod=Clip  InterpolateDimension=2  TableData=SimIn.Control.trim.B_lon_interp  SimulateUsing=Code generation
  Matrix Interpolation2 : simulink_extras/Additional Lookup Tables/Matrix Interpolation  InterpMethod=Linear  ExtrapMethod=Clip  InterpolateDimension=2  TableData=SimIn.Control.trim.Ki_lon_interp  SimulateUsing=Code generation
  Matrix Interpolation3 : simulink_extras/Additional Lookup Tables/Matrix Interpolation  InterpMethod=Linear  ExtrapMethod=Clip  InterpolateDimension=2  TableData=SimIn.Control.trim.Kx_lon_interp  SimulateUsing=Code generation
  Matrix Interpolation4 : simulink_extras/Additional Lookup Tables/Matrix Interpolation  InterpMethod=Linear  ExtrapMethod=Clip  InterpolateDimension=2  TableData=SimIn.Control.trim.F_lon_interp  SimulateUsing=Code generation
  Matrix Interpolation5 : simulink_extras/Additional Lookup Tables/Matrix Interpolation  InterpMethod=Linear  ExtrapMethod=Clip  InterpolateDimension=2  TableData=SimIn.Control.trim.Ap_lon_interp  SimulateUsing=Code generation
  Matrix Interpolation6 : simulink_extras/Additional Lookup Tables/Matrix Interpolation  InterpMethod=Linear  ExtrapMethod=Clip  InterpolateDimension=2  TableData=SimIn.Control.trim.Bp_lon_interp  SimulateUsing=Code generation
  Matrix Interpolation8 : simulink_extras/Additional Lookup Tables/Matrix Interpolation  InterpMethod=Linear  ExtrapMethod=Clip  InterpolateDimension=2  TableData=SimIn.Control.trim.G_lon_interp  SimulateUsing=Code generation
  ctrl_sys_lon : Outport
  wires:
  f2/1 -> Matrix Interpolation6/4, Matrix Interpolation5/4, Matrix Interpolation16/4, Matrix Interpolation15/4, Matrix Interpolation14/4, Matrix Interpolation13/4, Matrix Interpolation8/4, Matrix Interpolation4/4, Matrix Interpolation12/4, Matrix Interpolation3/4, Matrix Interpolation2/4
  Bus Creator/1 -> ctrl_sys_lon/1  "ctrl_sys_lon"
  Matrix Interpolation12/1 -> Bus Creator/3  "Kv"
  Matrix Interpolation15/1 -> Bus Creator/8  "W"
  Matrix Interpolation5/1 -> Bus Creator/10  "Ap"
  Matrix Interpolation4/1 -> Bus Creator/4  "F"
  Matrix Interpolation14/1 -> Bus Creator/7  "Cv"
  Matrix Interpolation2/1 -> Bus Creator/1  "Ki"
  Matrix Interpolation16/1 -> Bus Creator/9  "B"
  Matrix Interpolation8/1 -> Bus Creator/5  "G"
  Matrix Interpolation13/1 -> Bus Creator/6  "C"
  Matrix Interpolation3/1 -> Bus Creator/2  "Kx"
  k1/1 -> Matrix Interpolation16/1, Matrix Interpolation6/1, Matrix Interpolation5/1, Matrix Interpolation15/1, Matrix Interpolation14/1, Matrix Interpolation13/1, Matrix Interpolation8/1, Matrix Interpolation4/1, Matrix Interpolation12/1, Matrix Interpolation3/1, Matrix Interpolation2/1
  k2/1 -> Matrix Interpolation6/3, Matrix Interpolation5/3, Matrix Interpolation16/3, Matrix Interpolation15/3, Matrix Interpolation14/3, Matrix Interpolation13/3, Matrix Interpolation8/3, Matrix Interpolation4/3, Matrix Interpolation12/3, Matrix Interpolation3/3, Matrix Interpolation2/3
  Matrix Interpolation6/1 -> Bus Creator/11  "Bp"
  f1/1 -> Matrix Interpolation6/2, Matrix Interpolation5/2, Matrix Interpolation16/2, Matrix Interpolation15/2, Matrix Interpolation14/2, Matrix Interpolation13/2, Matrix Interpolation8/2, Matrix Interpolation4/2, Matrix Interpolation12/2, Matrix Interpolation3/2, Matrix Interpolation2/2

== system Baseline/L1 Adaptive/Lateral L1/Adaptation Law ==
  x_hat : Inport
  x : Inport  Port=2
  As : Inport  Port=3
  Constant : Constant  Value=SimIn.Environment.Turbulence.dT
  MATLAB Function : MATLAB Function  TreatAsAtomicUnit=on
  Matrix Multiply : Product  Multiplication=Matrix(*)
  Subtract : Sum  Inputs=+-
  sigma_hat : Outport
  wires:
  Subtract/1 -> Matrix Multiply/2
  MATLAB Function/1(Ka) -> Matrix Multiply/1
  Matrix Multiply/1 -> sigma_hat/1
  [Ts] -> MATLAB Function/2(Ts)
  [As] -> MATLAB Function/1(As)
  As/1 -> [As]
  Constant/1 -> [Ts]
  x/1 -> Subtract/2
  x_hat/1 -> Subtract/1

== system Baseline/L1 Adaptive/Lateral L1/Control Law ==
  sigma_hat : Inport
  Demux : Demux  Outputs=3
  Gain : Gain  Gain=-1
  Mux : Mux  Inputs=3
  Transfer Fcn : TransferFcn  Numerator=[L1_LPF_bw(4)^2]  Denominator=[1 L1_LPF_bw(4)*sqrt(2) L1_LPF_bw(4)^2]
  Transfer Fcn3 : TransferFcn  Numerator=[L1_LPF_bw(6)^2]  Denominator=[1 L1_LPF_bw(6)*sqrt(2) L1_LPF_bw(6)^2]
  Transfer Fcn4 : TransferFcn  Numerator=[L1_LPF_bw(5)^2]  Denominator=[1 L1_LPF_bw(5)*sqrt(2) L1_LPF_bw(5)^2]
  Out1 : Outport
  wires:
  Gain/1 -> Out1/1
  Mux/1 -> Gain/1
  sigma_hat/1 -> Demux/1
  Transfer Fcn/1 -> Mux/1
  Demux/1 -> Transfer Fcn/1
  Transfer Fcn4/1 -> Mux/2
  Demux/2 -> Transfer Fcn4/1
  Demux/3 -> Transfer Fcn3/1
  Transfer Fcn3/1 -> Mux/3

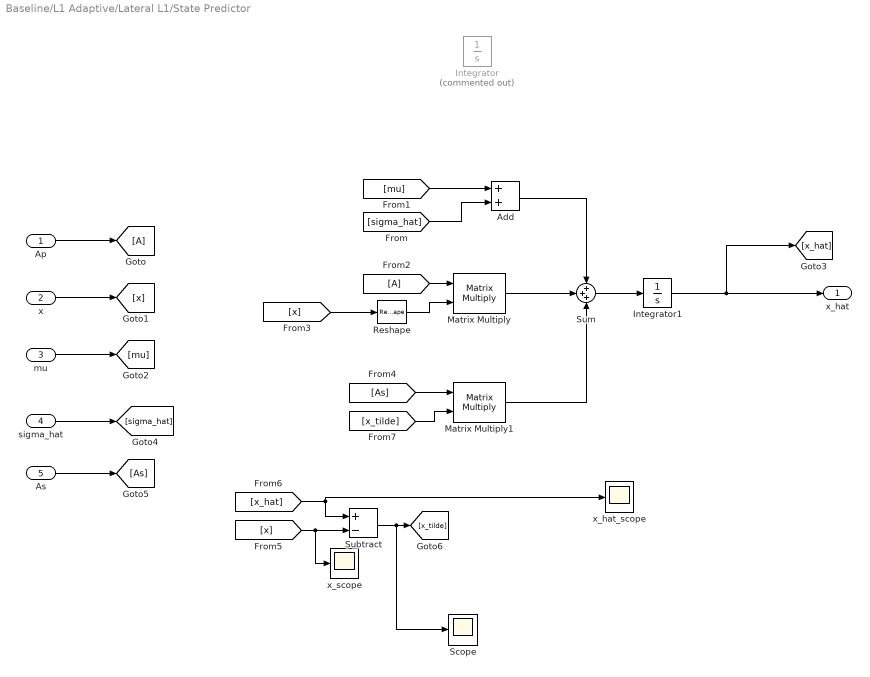
== system Baseline/L1 Adaptive/Lateral L1/State Predictor ==
  Ap : Inport
  x : Inport  Port=2
  mu : Inport  Port=3
  sigma_hat : Inport  Port=4
  As : Inport  Port=5
  Add : Sum
  From2 : From
  Goto : Goto
  Integrator : Integrator  Commented=on  InitialCondition=[SimPar.EOM.Vel_bEb; SimPar.EOM.Omeg_BIb; SimPar.EOM.Pos_bii; SimPar.EOM.Q_i2b]  LimitOutput=on  UpperSaturationLimit=[inf; inf; inf; 10; 10; 10; inf; inf; inf; 1; 1; 1; 1]  LowerSaturationLimit=-[inf; inf; inf; 10; 10; 10; inf; inf; inf; 1; 1; 1; 1]  ContinuousStateAttributes='EOMStates'
  Integrator1 : Integrator  InitialCondition=zeros(3,1)
  Matrix Multiply : Product  Multiplication=Matrix(*)
  Matrix Multiply1 : Product  Multiplication=Matrix(*)
  Reshape : Reshape  OutputDimensionality=Column vector (2-D)
  Scope : Scope
      settings: ActiveDisplayYMinimum=-0.065987635715359039  ActiveDisplayYMaximum=0.11704385068674639  DataLoggingVariableName=ScopeData7
  Subtract : Sum  Inputs=+-
  Sum : Sum  Inputs=+++
  x_hat_scope : Scope
      settings: ActiveDisplayYMinimum=-12.893051205580424  ActiveDisplayYMaximum=26.883895053159652  DataLoggingVariableName=ScopeData8
  x_scope : Scope
      settings: ActiveDisplayYMinimum=-8.15273768204296  ActiveDisplayYMaximum=4.9390300189148082  DataLoggingVariableName=ScopeData9
  x_hat : Outport
  wires:
  [x] -> Reshape/1
  Reshape/1 -> Matrix Multiply/2
  [x_tilde] -> Matrix Multiply1/2
  Subtract/1 -> [x_tilde], Scope/1
  [x_hat] -> Subtract/1, x_hat_scope/1
  [x] -> Subtract/2, x_scope/1
  [As] -> Matrix Multiply1/1
  Matrix Multiply1/1 -> Sum/3
  As/1 -> [As]
  Add/1 -> Sum/1
  [sigma_hat] -> Add/2
  [mu] -> Add/1
  From2/1 -> Matrix Multiply/1
  sigma_hat/1 -> [sigma_hat]
  Matrix Multiply/1 -> Sum/2
  Sum/1 -> Integrator1/1
  Integrator1/1 -> [x_hat], x_hat/1
  mu/1 -> [mu]
  x/1 -> [x]
  Ap/1 -> Goto/1

== system Baseline/L1 Adaptive/Longitudinal L1/Adaptation Law ==
  x_hat : Inport
  x : Inport  Port=2
  As : Inport  Port=3
  Constant : Constant  Value=SimIn.Environment.Turbulence.dT
  Demux : Demux  Outputs=3
  Gain : Gain  Gain=-1
  MATLAB Function : MATLAB Function  TreatAsAtomicUnit=on
  Matrix Multiply : Product  Multiplication=Matrix(*)
  Mux : Mux  Inputs=3
  Scope : Scope
      settings: ActiveDisplayYMinimum=-0.036620080657833093  ActiveDisplayYMaximum=0.037036557321583452  DataLoggingVariableName=ScopeData14
  Subtract : Sum  Inputs=+-
  sigma_hat : Outport
  wires:
  Mux/1 -> Scope/1
  Gain/1 -> Demux/1
  Demux/3 -> Mux/3  "sigma hat 3"
  Demux/2 -> Mux/2  "sigma hat 2"
  Demux/1 -> Mux/1  "sigma hat 1"
  Matrix Multiply/1 -> Gain/1, sigma_hat/1
  Constant/1 -> [Ts]
  Subtract/1 -> Matrix Multiply/2
  MATLAB Function/1(Ka) -> Matrix Multiply/1
  [Ts] -> MATLAB Function/2(Ts)
  [As] -> MATLAB Function/1(As)
  As/1 -> [As]
  x/1 -> Subtract/2
  x_hat/1 -> Subtract/1

== system Baseline/L1 Adaptive/Longitudinal L1/Control Law ==
  sigma_hat : Inport
  Demux : Demux  Outputs=3
  Gain : Gain  Gain=-1
  Mux : Mux  Inputs=3
  Transfer Fcn : TransferFcn  Numerator=[L1_LPF_bw(1)^2]  Denominator=[1 L1_LPF_bw(1)*sqrt(2) L1_LPF_bw(1)^2]
  Transfer Fcn3 : TransferFcn  Numerator=[L1_LPF_bw(3)^2]  Denominator=[1 L1_LPF_bw(3)*sqrt(2) L1_LPF_bw(3)^2]
  Transfer Fcn4 : TransferFcn  Numerator=[L1_LPF_bw(2)^2]  Denominator=[1 L1_LPF_bw(2)*sqrt(2) L1_LPF_bw(2)^2]
  Out1 : Outport
  wires:
  Gain/1 -> Out1/1
  Mux/1 -> Gain/1
  Transfer Fcn/1 -> Mux/1
  Demux/1 -> Transfer Fcn/1
  sigma_hat/1 -> Demux/1
  Transfer Fcn3/1 -> Mux/3
  Demux/3 -> Transfer Fcn3/1
  Demux/2 -> Transfer Fcn4/1
  Transfer Fcn4/1 -> Mux/2

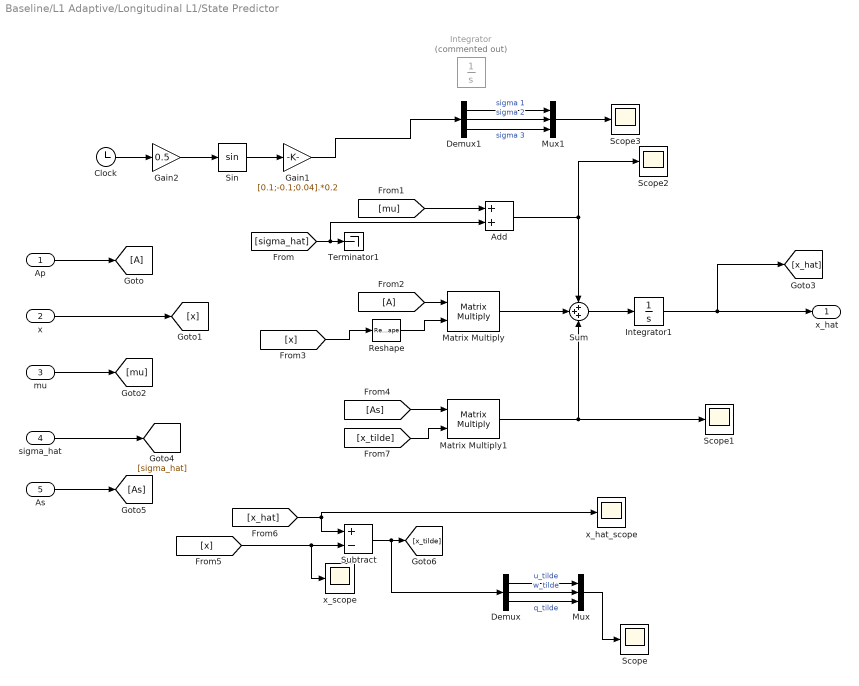
== system Baseline/L1 Adaptive/Longitudinal L1/State Predictor ==
  Ap : Inport
  x : Inport  Port=2
  mu : Inport  Port=3
  sigma_hat : Inport  Port=4
  As : Inport  Port=5
  Add : Sum
  Clock : Clock
  Demux : Demux  Outputs=3
  Demux1 : Demux  Outputs=3
  From2 : From
  Gain1 : Gain  Gain=[0.1;-0.1;0.04].*0.2
  Gain2 : Gain  Gain=0.5
  Goto : Goto
  Integrator : Integrator  Commented=on  InitialCondition=[SimPar.EOM.Vel_bEb; SimPar.EOM.Omeg_BIb; SimPar.EOM.Pos_bii; SimPar.EOM.Q_i2b]  LimitOutput=on  UpperSaturationLimit=[inf; inf; inf; 10; 10; 10; inf; inf; inf; 1; 1; 1; 1]  LowerSaturationLimit=-[inf; inf; inf; 10; 10; 10; inf; inf; inf; 1; 1; 1; 1]  ContinuousStateAttributes='EOMStates'
  Integrator1 : Integrator  InitialCondition=zeros(3,1)
  Matrix Multiply : Product  Multiplication=Matrix(*)
  Matrix Multiply1 : Product  Multiplication=Matrix(*)
  Mux : Mux  Inputs=3
  Mux1 : Mux  Inputs=3
  Reshape : Reshape  OutputDimensionality=Column vector (2-D)
  Scope{,1..3} (4 alike) : Scope
      Scope settings: ActiveDisplayYMinimum=-0.15796209283513146  ActiveDisplayYMaximum=0.57310689920390157  DataLoggingVariableName=ScopeData7
      Scope1 settings: ActiveDisplayYMinimum=-1  ActiveDisplayYMaximum=1  DataLoggingVariableName=ScopeData10
      Scope2 settings: ActiveDisplayYMinimum=-1  ActiveDisplayYMaximum=1  DataLoggingVariableName=ScopeData13
      Scope3 settings: ActiveDisplayYMinimum=-0.024999999845933065  ActiveDisplayYMaximum=0.024999999845933065  DataLoggingVariableName=ScopeData15
  Sin : Trigonometry
  Subtract : Sum  Inputs=+-
  Sum : Sum  Inputs=+++
  Terminator1 : Terminator
  x_hat_scope : Scope
      settings: ActiveDisplayYMinimum=-166.51310284407202  ActiveDisplayYMaximum=139.36129073032717  DataLoggingVariableName=ScopeData8
  x_scope : Scope
      settings: ActiveDisplayYMinimum=-1  ActiveDisplayYMaximum=1  DataLoggingVariableName=ScopeData9
  x_hat : Outport
  wires:
  Mux/1 -> Scope/1
  Demux/3 -> Mux/3  "q_tilde"
  Demux/2 -> Mux/2  "w_tilde"
  Demux/1 -> Mux/1  "u_tilde"
  sigma_hat/1 -> [sigma_hat]
  x/1 -> [x]
  Reshape/1 -> Matrix Multiply/2
  [x_tilde] -> Matrix Multiply1/2
  Subtract/1 -> [x_tilde], Demux/1
  [x_hat] -> Subtract/1, x_hat_scope/1
  [x] -> Subtract/2, x_scope/1
  [As] -> Matrix Multiply1/1
  Matrix Multiply1/1 -> Sum/3, Scope1/1
  As/1 -> [As]
  Add/1 -> Sum/1, Scope2/1
  [mu] -> Add/1
  [x] -> Reshape/1
  From2/1 -> Matrix Multiply/1
  Matrix Multiply/1 -> Sum/2
  Sum/1 -> Integrator1/1
  Integrator1/1 -> [x_hat], x_hat/1
  mu/1 -> [mu]
  Ap/1 -> Goto/1
  Clock/1 -> Gain2/1
  Sin/1 -> Gain1/1
  [sigma_hat] -> Add/2, Terminator1/1
  Gain2/1 -> Sin/1
  Mux1/1 -> Scope3/1
  Demux1/1 -> Mux1/1  "sigma 1"
  Gain1/1 -> Demux1/1
  Demux1/3 -> Mux1/3  "sigma 3"
  Demux1/2 -> Mux1/2  "sigma 2"

== matlab function Baseline/Scheduled Parameters/Smart_Interpolation ==
  data: u input; u_out output
function u_out = fcn(u)

% This function is used to limit interpolation for three portions of the
% flight envelope: 1) Below zero knots, 2) After the end of transition
% (90 kts) and before cruise (100 knots) and 3) above the last trim map
% point (130 knots)

ft2kts = 0.3048/1852.0*3600; % Conversion factor of ft/sec to knots (derived from setUnits values)
kts2ft = 1/ft2kts; % Conversion factor from knots to ft/sec
if u < 0* kts2ft; % SimIn.Control.trim.UH(1)
    u_out = 0*kts2ft; % SimIn.Control.trim.UH(1);
% elseif u>90*kts2ft && u<100*kts2ft
%     u_out = 100*kts2ft;
elseif u>130*kts2ft % SimIn.Control.trim.UH(end)
    u_out = 130*kts2ft; % SimIn.Control.trim.UH(end)
else
    u_out = u;
end

== matlab function Baseline/Pseudo Inverse Control Allocation/MATLAB Function ==
  data: M_lon input; u output; mdes_lon input; theta output; eng_max input; eng_min input; act_max input; act_min input
function [u, theta] = Limited_Allocation(M_lon, mdes_lon, eng_max, eng_min, act_max, act_min)

[u, theta] = Limited_Long_Cont_Alloc(M_lon, mdes_lon, eng_max, eng_min, act_max, act_min);

== matlab function Baseline/L1 Adaptive/Longitudinal L1/Adaptation Law/MATLAB Function ==
  data: As input; Ts input; Ka output
function Ka = fcn(As, Ts)

mat_exp = expm(As * Ts);
As_inv = pinv(As);

Ka = - pinv(As_inv * (mat_exp - eye(3))) * mat_exp;

end

== matlab function Baseline/L1 Adaptive/Lateral L1/Adaptation Law/MATLAB Function ==
  data: As input; Ts input; Ka output
function Ka = fcn(As, Ts)

mat_exp = expm(As * Ts);
As_inv = pinv(As);

Ka = - pinv(As_inv * (mat_exp - eye(3))) * mat_exp;

end
